simulink model "gm_transmitter"  (R2020b)
settings: Solver=FixedStepDiscrete  StartTime=0.0  StopTime=100000  RelTol=1e-3
undefined symbols (not defined in the file or in its folder): message
libraries: hdlmdlgenlib x28, simulink x10, hdlsllib x9, dspsigops x8, dspmlti4 x2, whdlio x1
(part 2 of 2)

== system gm_transmitter/tran_dut/ldpc_encoder/address_calculator/addresses ==
  slot : Inport  OutDataTypeStr=uint8  PortDimensions=1  SampleTime=2.06577425218972
  counter : Inport  Port=2  OutDataTypeStr=fixdt(0, 9, 0)  PortDimensions=1  SampleTime=2.06577425218972
  q_factor : Inport  Port=3  OutDataTypeStr=uint8  PortDimensions=1  SampleTime=2.06577425218972
  addresses1 : MATLAB Function  TreatAsAtomicUnit=on  mask{bit_addresses=uint16([[0 6385 7901 14611 13389 11200 3252 5243 2504 2722 821 7374]; [1 11359 2698 357 13824 12772 7244 6752 15310 852 2001 11417]; [2 7862 7977 6321 13612 12197 14449 15137 13860 1708 6399 13444]; [3 1560 11804 6975 13292 3646 3812 8772 7306 5795 14327 7866]; [4 7626 11407 14599 9689 1628 2113 10809 9283 1230 15241 4870]; [5 1610 5699 15876 9446 12515 1400 6303 5411 14181 13925 7358]; [6 4059 8836 3405 7853 7992 15336 5970 10368 10278 9675 4651]; [7 4441 3963 9153 2109 12683 7459 12030 12221 629 15212 406]; [8 6007 8411 5771 3497 543 14202 875 9186 6235 13908 3563]; [9 3232 6625 4795 546 9781 2071 7312 3399 7250 4932 12652]; [10 8820 10088 11090 7069 6585 13134 10158 7183 488 7455 9238]; [11 1903 10818 119 215 7558 11046 10615 11545 14784 7961 15619]; [12 3655 8736 4917 15874 5129 2134 15944 14768 7150 2692 1469]; [13 8316 3820 505 8923 6757 806 7957 4216 15589 13244 2622]; [14 14463 4852 15733 3041 11193 12860 13673 8152 6551 15108 8758]; [15 3149 11981 16200 16200 16200 16200 16200 16200 16200 16200 16200]; [16 13416 6906 16200 16200 16200 16200 16200 16200 16200 16200 16200]; [17 13098 13352 16200 16200 16200 16200 16200 16200 16200 16200 16200]; [18 2009 14460 16200 16200 16200 16200 16200 16200 16200 16200 16200]; [19 7207 4314 16200 16200 16200 16200 16200 16200 16200 16200 16200]; [20 3312 3945 16200 16200 16200 16200 16200 16200 16200 16200 16200]; [21 4418 6248 16200 16200 16200 16200 16200 16200 16200 16200 16200]; [22 2669 13975 16200 16200 16200 16200 16200 16200 16200 16200 16200]; [23 7571 9023 16200 16200 16200 16200 16200 16200 16200 16200 16200]; [24 14172 2967 16200 16200 16200 16200 16200 16200 16200 16200 16200]; [25 7271 7138 16200 16200 16200 16200 16200 16200 16200 16200 16200]; [26 6135 13670 16200 16200 16200 16200 16200 16200 16200 16200 16200]; [27 7490 14559 16200 16200 16200 16200 16200 16200 16200 16200 16200]; [28 8657 2466 16200 16200 16200 16200 16200 16200 16200 16200 16200]; [29 8599 12834 16200 16200 16200 16200 16200 16200 16200 16200 16200]; [30 3470 3152 16200 16200 16200 16200 16200 16200 16200 16200 16200]; [31 13917 4365 16200 16200 16200 16200 16200 16200 16200 16200 16200]; [32 6024 13730 16200 16200 16200 16200 16200 16200 16200 16200 16200]; [33 10973 14182 16200 16200 16200 16200 16200 16200 16200 16200 16200]; [34 2464 13167 16200 16200 16200 16200 16200 16200 16200 16200 16200]; [35 5281 15049 16200 16200 16200 16200 16200 16200 16200 16200 16200]; [36 1103 1849 16200 16200 16200 16200 16200 16200 16200 16200 16200]; [37 2058 1069 16200 16200 16200 16200 16200 16200 16200 16200 16200]; [38 9654 6095 16200 16200 16200 16200 16200 16200 16200 16200 16200]; [39 14311 7667 16200 16200 16200 16200 16200 16200 16200 16200 16200]; [40 15617 8146 16200 16200 16200 16200 16200 16200 16200 16200 16200]; [41 4588 11218 16200 16200 16200 16200 16200 16200 16200 16200 16200]; [42 13660 6243 16200 16200 16200 16200 16200 16200 16200 16200 16200]; [43 8578 7874 16200 16200 16200 16200 16200 16200 16200 16200 16200]; [44 11741 2686 16200 16200 16200 16200 16200 16200 16200 16200 16200]; [0 1022 1264 16200 16200 16200 16200 16200 16200 16200 16200 16200]; [1 12604 9965 16200 16200 16200 16200 16200 16200 16200 16200 16200]; [2 8217 2707 16200 16200 16200 16200 16200 16200 16200 16200 16200]; [3 3156 11793 16200 16200 16200 16200 16200 16200 16200 16200 16200]; [4 354 1514 16200 16200 16200 16200 16200 16200 16200 16200 16200]; [5 6978 14058 16200 16200 16200 16200 16200 16200 16200 16200 16200]; [6 7922 16079 16200 16200 16200 16200 16200 16200 16200 16200 16200]; [7 15087 12138 16200 16200 16200 16200 16200 16200 16200 16200 16200]; [8 5053 6470 16200 16200 16200 16200 16200 16200 16200 16200 16200]; [9 12687 14932 16200 16200 16200 16200 16200 16200 16200 16200 16200]; [10 15458 1763 16200 16200 16200 16200 16200 16200 16200 16200 16200]; [11 8121 1721 16200 16200 16200 16200 16200 16200 16200 16200 16200]; [12 12431 549 16200 16200 16200 16200 16200 16200 16200 16200 16200]; [13 4129 7091 16200 ...(+5412 chars)]]);, num_parity_bits=16200}
  addresses : Outport  VectorParamsAs1DForOutWhenUnconnected=off
  wires:
  addresses1/1(addresses) -> addresses/1
  slot/1 -> addresses1/1(slot)
  counter/1 -> addresses1/2(counter)
  q_factor/1 -> addresses1/3(q_factor)

== matlab function gm_transmitter/tran_dut/bit_mapping/angle_selector/angle_selector ==
  settings: fimath=fimath('RoundingMethod', 'Floor','OverflowAction', 'Wrap','ProductMode', 'FullPrecision', 'SumMode', 'FullPrecision')
  data: input input; phase output
function phase = phase_selector(input)
%#codegen
% Receives a bit sequence and returns the angle in radians of the
% corresponding 8-psk constellation symbol. Gray encoding is used as stated
% in the DVB-S2 standard.
    tmp = 0; % Start at phase 0
    if(input == 1)
        tmp=0;
    elseif(input == 0)
        tmp=45;
    elseif(input == 4)
        tmp=90;
    elseif(input == 6)
        tmp=135;
    elseif(input == 2)
        tmp=180;
    elseif(input == 3)
        tmp=225;
    elseif(input == 7)
        tmp=270;
    elseif(input == 5)
        tmp=315;
    end
    % 9 bits necessary to represent 360 degrees.
    phase = fi(tmp, 0, 23, 14, hdlfimath);

== matlab function gm_transmitter/tran_dut/ldpc_encoder/address_calculator/addresses/addresses1 ==
  settings: fimath=fimath('RoundingMethod', 'Floor','OverflowAction', 'Wrap','ProductMode', 'FullPrecision', 'SumMode', 'FullPrecision')
  data: slot input; counter input; q_factor input; addresses output uint16; bit_addresses parameter uint16; num_parity_bits parameter uint16
function addresses = address_generator(slot, counter, q_factor, bit_addresses, num_parity_bits)
%#codegen
buffer = uint16(bit_addresses(slot, :) + counter*q_factor);
addresses = buffer - uint16(num_parity_bits) .* uint16(buffer >= num_parity_bits);

== matlab function gm_transmitter/tran_dut/ldpc_encoder/MATLAB Function/MATLAB Function ==
  settings: fimath=fimath('RoundingMethod', 'Floor','OverflowAction', 'Wrap','ProductMode', 'FullPrecision', 'SumMode', 'FullPrecision')
  data: parity_in input fixdt(0,1,0); parity_out output fixdt(0,1,0); addresses input; input_bit input
function parity_out = select_and_xor(parity_in, addresses, input_bit)
%#codegen

parity_out = parity_in;
parity_out(addresses+1) = xor(parity_in(addresses+1), input_bit);

== matlab function gm_transmitter/tran_dut/ldpc_encoder/p2s/p2s ==
  settings: fimath=fimath('RoundingMethod', 'Floor','OverflowAction', 'Wrap','ProductMode', 'FullPrecision', 'SumMode', 'FullPrecision')
  data: parallel_in input; serial_out output fixdt(0,1,0); enable input; input_length parameter uint16; valid output
function [serial_out, valid] = p2s_buffer(parallel_in, enable, input_length)
%#codegen

state_iddle   = 0;
state_reading = 1;

persistent moore_state_machine;
if isempty(moore_state_machine)
    moore_state_machine = fi(0, 0, 1, 0);
end

persistent counter;
if isempty(counter)
    counter = fi(1, 0, 16, 0);
end

persistent buffer;
if isempty(buffer)
    buffer = parallel_in;
end

switch moore_state_machine
    case state_iddle
        serial_out = fi(0, 0, 1, 0);
        valid      = fi(0, 0, 1, 0);
        if enable
            moore_state_machine(1) = state_reading;
            buffer = parallel_in;
            serial_out          = buffer(counter);
            counter             = fi(counter + 1, 0, 16, 0);
            valid               = fi(1, 0, 1, 0);
        end
    case state_reading
        serial_out = buffer(counter);
        counter    = fi(counter + 1, 0, 16, 0);
        valid      = fi(1, 0, 1, 0);
        if(counter > input_length)
            moore_state_machine(1) = state_iddle;
        end
    otherwise
        serial_out = fi(0, 0, 1, 0);
        valid      = fi(0, 0, 1, 0);
end

== matlab function gm_transmitter/tran_dut/bch_encoder/output_mask/output_mask ==
  settings: fimath=fimath('RoundingMethod', 'Floor','OverflowAction', 'Wrap','ProductMode', 'FullPrecision', 'SumMode', 'FullPrecision')
  data: bit_in input; mask output
function mask = bitmask(bit_in)
%#codegen

if bit_in
    mask = fi(ones(192, 1), 0, 1, 0);
else
    mask = fi(zeros(192, 1), 0, 1, 0);
end

== matlab function gm_transmitter/tran_dut/bch_encoder/p2s/p2s ==
  settings: fimath=fimath('RoundingMethod', 'Floor','OverflowAction', 'Wrap','ProductMode', 'FullPrecision', 'SumMode', 'FullPrecision')
  data: parallel_in input; serial_out output fixdt(0,1,0); enable input; input_length parameter uint16; valid output
function [serial_out, valid] = p2s_buffer(parallel_in, enable, input_length)
%#codegen

state_iddle    = 0;
state_reading  = 1;

persistent moore_state_machine;
if isempty(moore_state_machine)
    moore_state_machine = fi(0, 0, 1, 0);
end

persistent counter;
if isempty(counter)
    counter = fi(1, 0, 16, 0);
end

persistent buffer;
if isempty(buffer)
    buffer = parallel_in;
end

switch moore_state_machine
    case state_iddle
        serial_out = fi(0, 0, 1, 0);
        valid      = fi(0, 0, 1, 0);
        if enable
            moore_state_machine(1) = state_reading;
            buffer = parallel_in;
            serial_out          = buffer(input_length+1-counter);
            valid      = fi(1, 0, 1, 0);
            counter             = fi(counter + 1, 0, 16, 0);
        end
    case state_reading
        serial_out = buffer(input_length+1-counter);
        counter    = fi(counter + 1, 0, 16, 0);
        valid      = fi(1, 0, 1, 0);
        if(counter > input_length)
            counter = fi(1, 0, 16, 0);
            moore_state_machine(1) = state_iddle;
        end
    otherwise
        serial_out = fi(0, 0, 1, 0);
        valid      = fi(0, 0, 1, 0);
end

== matlab function gm_transmitter/tran_dut/bch_encoder/registers/registers ==
  settings: fimath=fimath('RoundingMethod', 'Floor','OverflowAction', 'Wrap','ProductMode', 'FullPrecision', 'SumMode', 'FullPrecision')
  data: registers_in input; out output fixdt(0,1,0) size=1; registers_out output fixdt(0,1,0) size=192
function [out, registers_out] = state_registers(registers_in)
%#codegen

persistent lfsr;
if isempty(lfsr)
    lfsr = fi(zeros(192, 1), 0, 1, 0);
else
    lfsr = registers_in;
end
out = lfsr(192);
registers_out = lfsr;

== matlab function gm_transmitter/tran_dut/bch_encoder/shift_and_xor/shift_and_xor ==
  settings: fimath=fimath('RoundingMethod', 'Floor','OverflowAction', 'Wrap','ProductMode', 'FullPrecision', 'SumMode', 'FullPrecision')
  data: input_bit input; registers_out output fixdt(0,1,0); registers_in input; flag input
function registers_out = shift_and_xor(input_bit, registers_in, flag)
%#codegen

buffer = [input_bit; registers_in(1:192-1)];
registers_out = fi(xor(buffer, flag), 0, 1, 0);
